simulink model "maglev"  (R2018b)
settings: Solver=VariableStepAuto  StartTime=0.0  StopTime=0  RelTol=1e-9
values from neighbouring files (symbols this model uses):
  A = []    [getBestQ.m]    (also in hw4.m = [0 1; 2*g/xeq 0])
  B = [0; -2*g/ieq]    [getBestQ.m]    (also in hw4.m)
  ieq = kff*xeq    [getBestQ.m]    (also in hw4.m)
  K = lqr(A, B, diag([10 1]),1)    [getBestQ.m]    (also in hw4.m = lqr(A,B,Q,R))
  param = [m; k; g]    [hw4.m]
  X0 = [14e-3; 0 ]    [hw4.m]
  xeq = 6e-3    (= 0.006)    [getBestQ.m]    (also in hw4.m)
undefined symbols (not defined in the file or in its folder): maglevDer
settings Model: Creator=Erivelton  LastModifiedBy=Erivelton

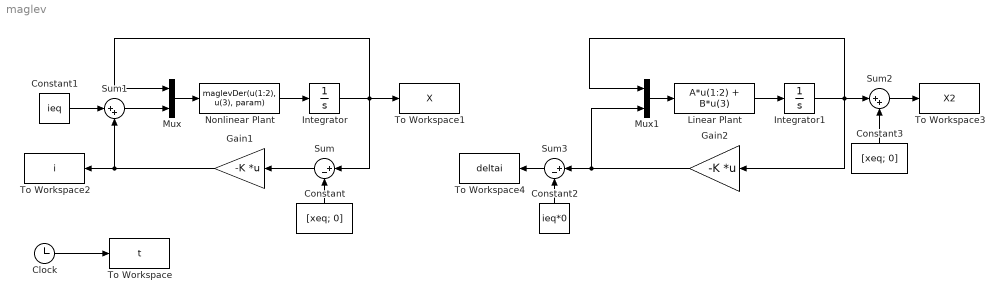
== system maglev ==
  Clock : Clock
  Constant : Constant  Value=[xeq; 0]
  Constant1 : Constant  Value=ieq
  Constant2 : Constant  Value=ieq*0
  Constant3 : Constant  Value=[xeq; 0]
  Gain1 : Gain  Gain=-K  Multiplication=Matrix(K*u) (u vector)
  Gain2 : Gain  Gain=-K  Multiplication=Matrix(K*u) (u vector)
  Integrator : Integrator  InitialCondition=X0
  Integrator1 : Integrator  InitialCondition=X0-[xeq; 0]
  Linear Plant : MATLABFcn  MATLABFcn=A*u(1:2) + B*u(3)  OutputDimensions=2
  Mux : Mux  Inputs=2
  Mux1 : Mux  Inputs=2
  Nonlinear Plant : MATLABFcn  MATLABFcn=maglevDer(u(1:2), u(3), param)
  Sum : Sum  Inputs=|+-
  Sum1 : Sum  Inputs=|++
  Sum2 : Sum  Inputs=|++
  Sum3 : Sum  Inputs=|+-
  To Workspace : ToWorkspace  VariableName=t  SampleTime=-1
  To Workspace1 : ToWorkspace  VariableName=X  SampleTime=-1
  To Workspace2 : ToWorkspace  VariableName=i  SampleTime=-1
  To Workspace3 : ToWorkspace  VariableName=X2  SampleTime=-1
  To Workspace4 : ToWorkspace  VariableName=deltai  SampleTime=-1
  wires:
  Sum/1 -> Gain1/1
  Mux/1 -> Nonlinear Plant/1
  Gain1/1 -> Sum1/2, To Workspace2/1
  Constant/1 -> Sum/2
  Integrator/1 -> Sum/1, Mux/1, To Workspace1/1
  Clock/1 -> To Workspace/1
  Nonlinear Plant/1 -> Integrator/1
  Sum1/1 -> Mux/2
  Constant1/1 -> Sum1/1
  Linear Plant/1 -> Integrator1/1
  Gain2/1 -> Mux1/2, Sum3/1
  Integrator1/1 -> Sum2/1, Gain2/1, Mux1/1
  Mux1/1 -> Linear Plant/1
  Sum2/1 -> To Workspace3/1
  Constant3/1 -> Sum2/2
  Sum3/1 -> To Workspace4/1
  Constant2/1 -> Sum3/2
